simulink model "axilite_template"  (R2018a)
settings: Solver=VariableStepAuto  StartTime=0.0  StopTime=300  RelTol=1e-3
undefined symbols (not defined in the file): AXI4, Lite
libraries: xbsIndex_r4 x4
settings Model: Creator=David Northcote  LastModifiedBy=David Northcote

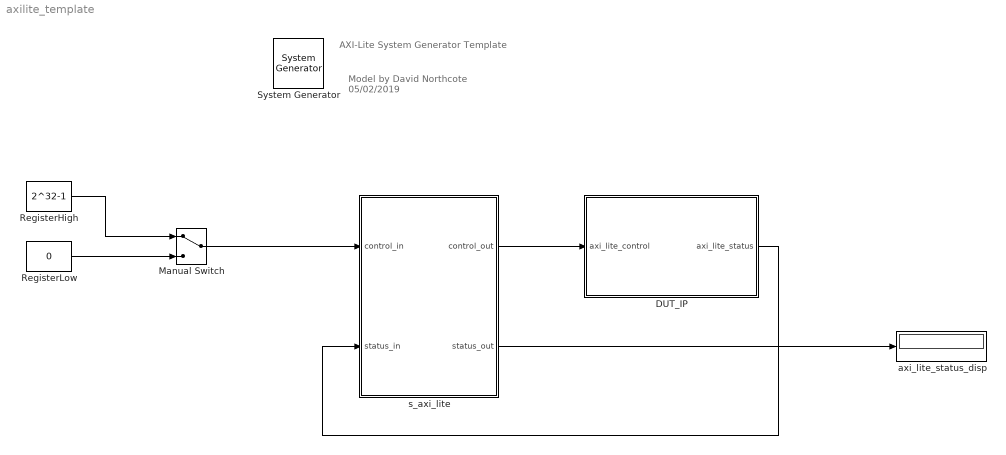
== system axilite_template ==
  note: Model by David Northcote
      | 05/02/2019
  note: AXI-Lite System Generator Template
  " System Generator" : xbsIndex_r4/ System Generator  Tag=genX  xilinxfamily=zynq  part=xc7z020  speed=-1  package=clg400  synthesis_tool=Vivado  clock_wrapper=Clock Enables  directory=./netlist  proj_type=Vivado  Synth_file=Vivado Synthesis Defaults  Impl_file=Vivado Implementation Defaults  testbench=off  simulink_period=1  sysclk_period=10  dcm_input_clock_period=10  incr_netlist=off  trim_vbits=Everywhere in SubSystem  dbl_ovrd=According to Block Masks  core_generation=According to Block Masks  run_coregen=off  deprecated_control=off  eval_field=0  block_type=sysgen
  DUT_IP : Subsystem
  Manual Switch : ManualSwitch
  RegisterHigh : Constant  Value=2^32-1  OutDataTypeStr=uint32  SampleTime=-1
  RegisterLow : Constant  Value=0  OutDataTypeStr=uint32  SampleTime=-1
  axi_lite_status_disp : Display
  s_axi_lite : Subsystem
  wires:
  Manual Switch/1 -> s_axi_lite/1(control_in)
  RegisterLow/1 -> Manual Switch/2
  RegisterHigh/1 -> Manual Switch/1
  s_axi_lite/2(status_out) -> axi_lite_status_disp/1
  s_axi_lite/1(control_out) -> DUT_IP/1(axi_lite_control)
  DUT_IP/1(axi_lite_status) -> s_axi_lite/2(status_in)

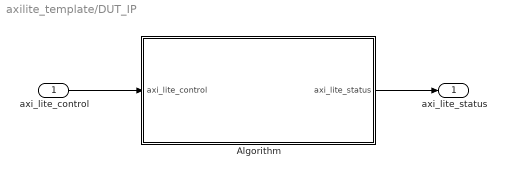
== system axilite_template/DUT_IP ==
  axi_lite_control : Inport
  Algorithm : Subsystem
  axi_lite_status : Outport
  wires:
  axi_lite_control/1 -> Algorithm/1(axi_lite_control)
  Algorithm/1(axi_lite_status) -> axi_lite_status/1

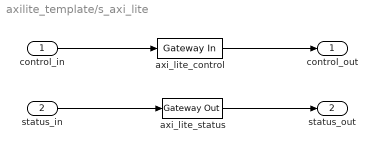
== system axilite_template/s_axi_lite ==
  control_in : Inport
  status_in : Inport  Port=2
  axi_lite_control : xbsIndex_r4/Gateway In  gui_display_data_type=Fixed-point  arith_type=Unsigned  n_bits=32  bin_pt=0  preci_type=Single  exp_width=8  frac_width=24  rows=1  columns=1  quantization="Round  (unbiased: +/- Inf)"  overflow=Saturate  period=1  UseAsADC=off  ADCChannel='1'  interface=AXI4-Lite  automatic_assignment=on  address_offset=hex2dec('00')  intf_name=''  intf_description=''  default_value=0  timing_constraint=None  locs_specified=off  LOCs={}  io_standard={}  inherit_from_input=off  hdl_port=on  dbl_ovrd=off  block_type=gatewayin
  axi_lite_status : xbsIndex_r4/Gateway Out  inherit_from_input=off  hdl_port=on  rows=1  columns=1  UseAsDAC=off  DACChannel='1'  interface=AXI4-Lite  automatic_assignment=on  address_offset=hex2dec('00')  intf_name=''  intf_description=''  timing_constraint=None  locs_specified=off  LOCs={}  io_standard={}  block_type=gatewayout
  control_out : Outport
  status_out : Outport  Port=2
  wires:
  axi_lite_control/1 -> control_out/1
  control_in/1 -> axi_lite_control/1
  status_in/1 -> axi_lite_status/1
  axi_lite_status/1 -> status_out/1

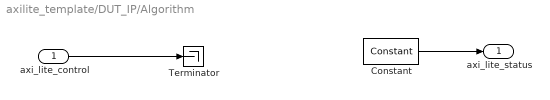
== system axilite_template/DUT_IP/Algorithm ==
  axi_lite_control : Inport
  Constant : xbsIndex_r4/Constant  const=0  gui_display_data_type=Fixed-point  arith_type=Unsigned  n_bits=32  bin_pt=0  preci_type=Single  exp_width=8  frac_width=24  explicit_period=on  period=1  equ=P=C  opselect=C  inp2=PCIN>>17  opr=+  inp1=P  carry=CIN  dbl_ovrd=off  block_type=constant
  Terminator : Terminator
  axi_lite_status : Outport
  wires:
  axi_lite_control/1 -> Terminator/1
  Constant/1 -> axi_lite_status/1
